simulink model "blockdemo2"  (Simulink 6.3)
settings: Solver=FixedStepDiscrete  StartTime=0.0  StopTime=10.0  FixedStep=1  RelTol=1e-3
InitFcn:
  | %% DSPBuilder Start
  | alt_dspbuilder_update_model(bdroot)
  | %% DSPBuilder End
libraries: allblocks_alteradspbuilder2 x13
settings Model: Creator=mjervis  LastModifiedBy=delphick
settings OptimizationCC: BooleanDataType=off  InlineInvariantSignals=on
settings DebuggingCC: SolverPrmCheckMsg=none
settings HardwareCC: TargetUnknown=on

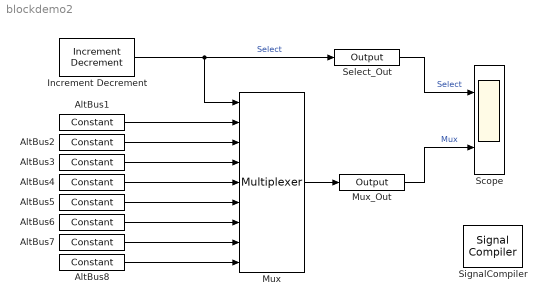
== system blockdemo2 ==
  AltBus1 : allblocks_alteradspbuilder2/Constant  mask_cst=1  BusType=Signed Integer  bwl=8  bwr=0  SpecifyClock=off
  AltBus2 : allblocks_alteradspbuilder2/Constant  mask_cst=2  BusType=Signed Integer  bwl=8  bwr=0  SpecifyClock=off
  AltBus3 : allblocks_alteradspbuilder2/Constant  mask_cst=3  BusType=Signed Integer  bwl=8  bwr=0  SpecifyClock=off
  AltBus4 : allblocks_alteradspbuilder2/Constant  mask_cst=4  BusType=Signed Integer  bwl=8  bwr=0  SpecifyClock=off
  AltBus5 : allblocks_alteradspbuilder2/Constant  mask_cst=5  BusType=Signed Integer  bwl=8  bwr=0  SpecifyClock=off
  AltBus6 : allblocks_alteradspbuilder2/Constant  mask_cst=6  BusType=Signed Integer  bwl=8  bwr=0  SpecifyClock=off
  AltBus7 : allblocks_alteradspbuilder2/Constant  mask_cst=7  BusType=Signed Integer  bwl=8  bwr=0  SpecifyClock=off
  AltBus8 : allblocks_alteradspbuilder2/Constant  mask_cst=8  BusType=Signed Integer  bwl=8  bwr=0  SpecifyClock=off
  Increment Decrement : allblocks_alteradspbuilder2/Increment Decrement  BusType=Unsigned Integer  bwl=8  bwr=0  SpecifyClock=off  clr_value=0  direction=Increment  phase_selection=1  use_ena=off  use_sclr=off
  Mux : allblocks_alteradspbuilder2/Multiplexer  numInputs=8  pipeline=0  oneHot=off  use_ena=off  use_aclr=off
  Mux_Out : allblocks_alteradspbuilder2/Output  iofile=C:\workspace_clean\Documentation\DesignExamples\Tutorials\UnitBlocks\GateAndControl\Multiplexer\tb_blockdemo2\blockdemo2_Mux_Out.capture  BusType=Signed Integer  bwl=14  bwr=0  PORTTYPE=Output
  Scope : Scope  NumInputPorts=2
      settings: YMin=-2~-2  YMax=10~10
  Select_Out : allblocks_alteradspbuilder2/Output  iofile=C:\workspace_clean\Documentation\DesignExamples\Tutorials\UnitBlocks\GateAndControl\Multiplexer\tb_blockdemo2\blockdemo2_Select_Out.capture  BusType=Unsigned Integer  bwl=8  bwr=0  PORTTYPE=Output
  SignalCompiler : allblocks_alteradspbuilder2/Signal Compiler  DeviceFamily=Stratix IV  DeviceName=AUTO  EnableSignalTap=off  SignalTapDepth=128  UseBoardBlock=off  StpUseDefaultClock=on  StpClock=clock
  wires:
  Increment Decrement/1 -> Mux/1, Select_Out/1  "Select"
  Mux_Out/1 -> Scope/2  "Mux"
  AltBus1/1 -> Mux/2
  AltBus2/1 -> Mux/3
  AltBus3/1 -> Mux/4
  AltBus4/1 -> Mux/5
  AltBus5/1 -> Mux/6
  AltBus6/1 -> Mux/7
  AltBus7/1 -> Mux/8
  AltBus8/1 -> Mux/9
  Mux/1 -> Mux_Out/1
  Select_Out/1 -> Scope/1  "Select"
